simulink library "fdclib2"  (Simulink 2.09)
values from neighbouring files (symbols this model uses):
  GM1 = [cbar b    S    Ix   Iy   Iz   Jxy  Jxz  Jyz  m]    [modbuild.m]

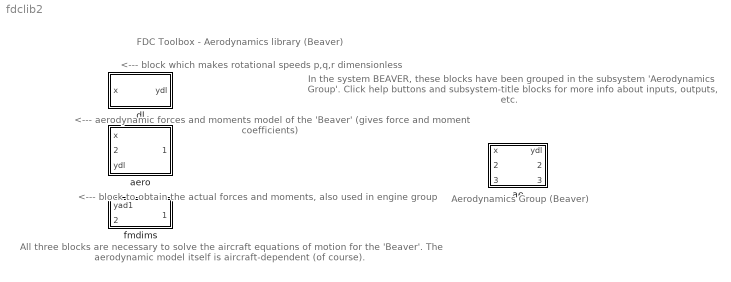
== system fdclib2 ==
  note: <--- block to obtain the actual
      | forces and moments, also used
      | in engine group
  note: <--- aerodynamic forces and moments
      | model of the 'Beaver' (gives force
      | and moment coefficients)
  note: <--- block which makes rotational
      | speeds p,q,r dimensionless
  note: All three blocks are necessary to solve the aircraft
      | equations of motion for the 'Beaver'. The aerodynamic
      | model itself is aircraft-dependent (of course).
  note: In the system BEAVER, these blocks have been
      | grouped in the subsystem 'Aerodynamics Group'.
      | Click help buttons and subsystem-title blocks
      | for more info about inputs, outputs, etc.
  note: Aerodynamics
      | Group (Beaver)
  note: FDC Toolbox - Aerodynamics library (Beaver)
  ae : Subsystem
  aero : Subsystem
      mask Type: Aeromod
      mask Description: Aerodynamic model of the DHC-2 'Beaver'.
      mask Help: eval('fdchelp aeromod')
      mask Display: disp('Aeromod\n(Beaver)')
  dl : Subsystem  mask(Dimless){cbar=GM1(1), b=GM1(2)}
      mask prompts: cbar "Mean aerodynamic chord [m]:"; b "Wing span [m]:"
      mask help: Dimensionless rotational velocities.
      mask Help: eval('fdchelp dimless')
      mask Display: disp('Dimless')
  fmdims : Subsystem  mask(FMdims){cbar=GM1(1), b=GM1(2), S=GM1(3)}
      mask prompts: cbar "Mean aerodynamic chord [m]:"; b "Wing span [m]:"; S "Wing surface [m^2]:"
      mask help:
      | Calculate forces and moments from
      | dimensionless coefficients.
      mask Help: eval('fdchelp fmdims')
      mask Display: disp('FMdims')

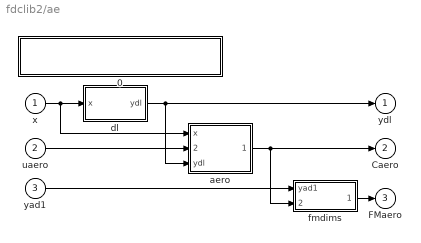
== system fdclib2/ae ==
  x : Inport  Port=1  PortWidth=-1  SampleTime=-1
  uaero : Inport  Port=2  PortWidth=-1  SampleTime=-1
  yad1 : Inport  Port=3  PortWidth=-1  SampleTime=-1
  0 : Subsystem
      settings: OpenFcn=fdchelp aerogrp
      mask Display: disp('AERODYNAMICS GROUP (level 3)\nM.O. Rauw')
  aero : Subsystem
      mask Type: Aeromod
      mask Description: Aerodynamic model of the DHC-2 'Beaver'.
      mask Help: eval('fdchelp aeromod')
      mask Display: disp('Aeromod\n(Beaver)')
  dl : Subsystem  mask(Dimless){cbar=GM1(1), b=GM1(2)}
      mask prompts: cbar "Mean aerodynamic chord [m]:"; b "Wing span [m]:"
      mask help: Dimensionless rotational velocities.
      mask Help: eval('fdchelp dimless')
      mask Display: disp('Dimless')
  fmdims : Subsystem  mask(FMdims){cbar=GM1(1), b=GM1(2), S=GM1(3)}
      mask prompts: cbar "Mean aerodynamic chord [m]:"; b "Wing span [m]:"; S "Wing surface [m^2]:"
      mask help:
      | Calculate forces and moments from
      | dimensionless coefficients.
      mask Help: eval('fdchelp fmdims')
      mask Display: disp('FMdims')
  ydl : Outport  Port=1  InitialOutput=0
  Caero : Outport  Port=2  InitialOutput=0
  FMaero : Outport  Port=3  InitialOutput=0
  wires:
  aero/1(Caero) -> Caero/1, fmdims/2(Force / moment coefficients)
  dl/1(ydl) -> ydl/1, aero/3(ydl)
  x/1 -> dl/1(x), aero/1(x)
  uaero/1 -> aero/2(uaero)
  yad1/1 -> fmdims/1(yad1)
  fmdims/1(Forces and moments) -> FMaero/1

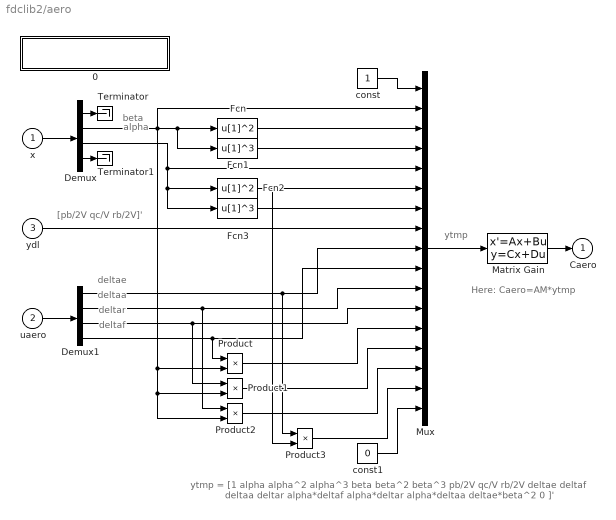
== system fdclib2/aero ==
  note: ytmp = [1  alpha  alpha^2  alpha^3  beta  beta^2  beta^3  pb/2V  qc/V  rb/2V  deltae
      | deltaf  deltaa  deltar  alpha*deltaf  alpha*deltar  alpha*deltaa  deltae*beta^2  0 ]'
  note: [pb/2V qc/V rb/2V]'
  note: beta
  note: deltae
  note: deltaa
  note: deltar
  note: deltaf
  note: alpha
  note: ytmp
  note: Here: Caero=AM*ytmp
  x : Inport  Port=1  PortWidth=-1  SampleTime=-1
  uaero : Inport  Port=2  PortWidth=-1  SampleTime=-1
  ydl : Inport  Port=3  PortWidth=-1  SampleTime=-1
  0 : Subsystem
      settings: OpenFcn=fdchelp aeromod
      mask Display: disp('AEROMOD\nM.O. Rauw, October 1997')
  Demux : Demux  Outputs=[1 1 1 9]
  Demux1 : Demux  Outputs=4
  Fcn : Fcn  Expr=u[1]^2
  Fcn1 : Fcn  Expr=u[1]^3
  Fcn2 : Fcn  Expr=u[1]^2
  Fcn3 : Fcn  Expr=u[1]^3
  Matrix Gain : StateSpace  A=A  B=B  C=C  D=D  X0=0  mask(Matrix Gain){@1=AM}
      mask prompts: @1 "Gain matrix:"
      mask help: Matrix Gain
      mask init:
      | A = []; B = []; C = []; D = @1;
      mask Help: This block implements an matrix gain.\nThe matrix dimensions must be in accordance\nwith the dimension of the inputvector.
      mask Display: disp('y = A*u')
  Mux : Mux  Inputs=[1 1 1 1 1 1 1 3 1 1 1 1 1 1 1 1 1]
  Product{,1..3} (4 alike) : Product  Inputs=2
  Terminator : Terminator
  Terminator1 : Terminator
  const : Constant  Value=1
  const1 : Constant  Value=0
  Caero : Outport  Port=1  InitialOutput=0
  wires:
  Demux/4 -> Terminator1/1
  Demux/1 -> Terminator/1
  const1/1 -> Mux/17
  const/1 -> Mux/1
  ydl/1 -> Mux/8
  Product3/1 -> Mux/16
  Product2/1 -> Mux/15
  Product1/1 -> Mux/14
  Demux1/1 -> Mux/9, Product3/1
  Fcn2/1 -> Mux/6, Product3/2
  Demux1/4 -> Mux/10, Product/1
  Demux/2 -> Mux/2, Fcn/1, Fcn1/1, Product/2, Product1/2, Product2/2
  Demux/3 -> Mux/5, Fcn2/1, Fcn3/1
  Demux1/2 -> Mux/11, Product2/1
  Demux1/3 -> Mux/12, Product1/1
  Product/1 -> Mux/13
  Fcn3/1 -> Mux/7
  uaero/1 -> Demux1/1
  Fcn1/1 -> Mux/4
  Fcn/1 -> Mux/3
  x/1 -> Demux/1
  Mux/1 -> Matrix Gain/1
  Matrix Gain/1 -> Caero/1

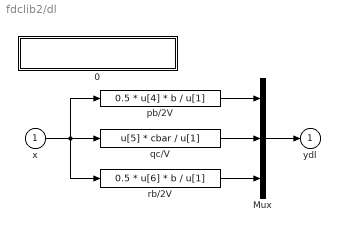
== system fdclib2/dl ==
  x : Inport  Port=1  PortWidth=-1  SampleTime=-1
  0 : Subsystem
      settings: OpenFcn=fdchelp dimless
      mask Display: disp('DIMLESS\nM.O. Rauw, October 1997')
  Mux : Mux  Inputs=3
  pb/2V : Fcn  Expr=0.5 * u[4] * b / u[1]
  qc/V : Fcn  Expr=u[5] * cbar / u[1]
  rb/2V : Fcn  Expr=0.5 * u[6] * b / u[1]
  ydl : Outport  Port=1  InitialOutput=0
  wires:
  pb/2V/1 -> Mux/1
  qc/V/1 -> Mux/2
  rb/2V/1 -> Mux/3
  Mux/1 -> ydl/1
  x/1 -> qc/V/1, rb/2V/1, pb/2V/1

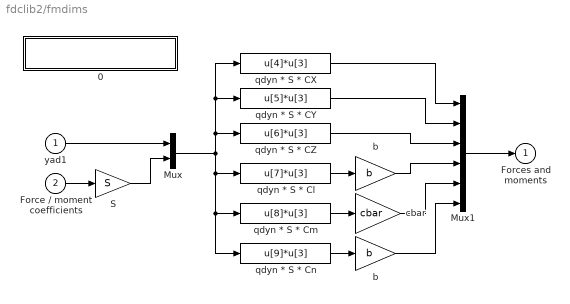
== system fdclib2/fmdims ==
  yad1 : Inport  Port=1  PortWidth=-1  SampleTime=-1
  Force / moment coefficients : Inport  Port=2  PortWidth=-1  SampleTime=-1
  0 : Subsystem
      settings: OpenFcn=fdchelp fmdims
      mask Display: disp('FMDIMS\nM.O. Rauw, October 1997')
  Mux : Mux  Inputs=[3 6]
  Mux1 : Mux  Inputs=6
  S : Gain  Gain=S
  b : Gain  Gain=b
  "b " : Gain  Gain=b
  cbar : Gain  Gain=cbar
  qdyn * S * CX : Fcn  Expr=u[4]*u[3]
  qdyn * S * CY : Fcn  Expr=u[5]*u[3]
  qdyn * S * CZ : Fcn  Expr=u[6]*u[3]
  qdyn * S * Cl : Fcn  Expr=u[7]*u[3]
  qdyn * S * Cm : Fcn  Expr=u[8]*u[3]
  qdyn * S * Cn : Fcn  Expr=u[9]*u[3]
  Forces and moments : Outport  Port=1  InitialOutput=0
  wires:
  Mux1/1 -> Forces and moments/1
  "b "/1 -> Mux1/6
  cbar/1 -> Mux1/5
  Force / moment coefficients/1 -> S/1
  Mux/1 -> qdyn * S * CZ/1, qdyn * S * CX/1, qdyn * S * CY/1, qdyn * S * Cl/1, qdyn * S * Cm/1, qdyn * S * Cn/1
  qdyn * S * Cl/1 -> b/1
  qdyn * S * Cm/1 -> cbar/1
  qdyn * S * Cn/1 -> "b "/1
  yad1/1 -> Mux/1
  qdyn * S * CX/1 -> Mux1/1
  qdyn * S * CY/1 -> Mux1/2
  S/1 -> Mux/2
  qdyn * S * CZ/1 -> Mux1/3
  b/1 -> Mux1/4

== system fdclib2/ae/0 ==

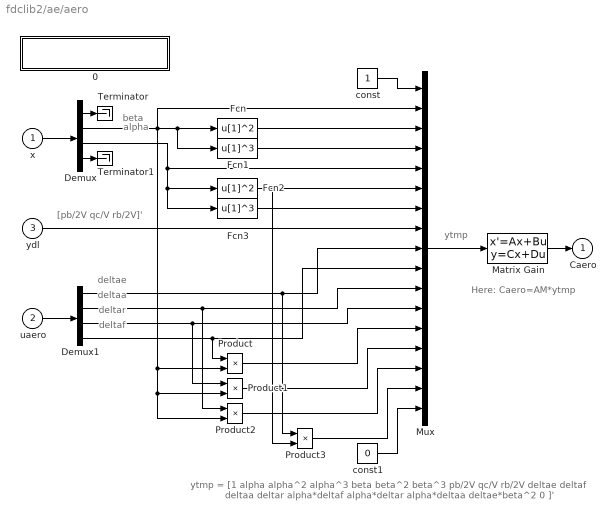
== system fdclib2/ae/aero ==
  note: ytmp = [1  alpha  alpha^2  alpha^3  beta  beta^2  beta^3  pb/2V  qc/V  rb/2V  deltae
      | deltaf  deltaa  deltar  alpha*deltaf  alpha*deltar  alpha*deltaa  deltae*beta^2  0 ]'
  note: [pb/2V qc/V rb/2V]'
  note: beta
  note: deltae
  note: deltaa
  note: deltar
  note: deltaf
  note: alpha
  note: ytmp
  note: Here: Caero=AM*ytmp
  x : Inport  Port=1  PortWidth=-1  SampleTime=-1
  uaero : Inport  Port=2  PortWidth=-1  SampleTime=-1
  ydl : Inport  Port=3  PortWidth=-1  SampleTime=-1
  0 : Subsystem
      settings: OpenFcn=fdchelp aeromod
      mask Display: disp('AEROMOD\nM.O. Rauw, October 1997')
  Demux : Demux  Outputs=[1 1 1 9]
  Demux1 : Demux  Outputs=4
  Fcn : Fcn  Expr=u[1]^2
  Fcn1 : Fcn  Expr=u[1]^3
  Fcn2 : Fcn  Expr=u[1]^2
  Fcn3 : Fcn  Expr=u[1]^3
  Matrix Gain : StateSpace  A=A  B=B  C=C  D=D  X0=0  mask(Matrix Gain){@1=AM}
      mask prompts: @1 "Gain matrix:"
      mask help: Matrix Gain
      mask init:
      | A = []; B = []; C = []; D = @1;
      mask Help: This block implements an matrix gain.\nThe matrix dimensions must be in accordance\nwith the dimension of the inputvector.
      mask Display: disp('y = A*u')
  Mux : Mux  Inputs=[1 1 1 1 1 1 1 3 1 1 1 1 1 1 1 1 1]
  Product{,1..3} (4 alike) : Product  Inputs=2
  Terminator : Terminator
  Terminator1 : Terminator
  const : Constant  Value=1
  const1 : Constant  Value=0
  Caero : Outport  Port=1  InitialOutput=0
  wires:
  Demux/4 -> Terminator1/1
  Demux/1 -> Terminator/1
  const1/1 -> Mux/17
  const/1 -> Mux/1
  ydl/1 -> Mux/8
  Product3/1 -> Mux/16
  Product2/1 -> Mux/15
  Product1/1 -> Mux/14
  Demux1/1 -> Mux/9, Product3/1
  Fcn2/1 -> Mux/6, Product3/2
  Demux1/4 -> Mux/10, Product/1
  Demux/2 -> Mux/2, Fcn/1, Fcn1/1, Product/2, Product1/2, Product2/2
  Demux/3 -> Mux/5, Fcn2/1, Fcn3/1
  Demux1/2 -> Mux/11, Product2/1
  Demux1/3 -> Mux/12, Product1/1
  Product/1 -> Mux/13
  Fcn3/1 -> Mux/7
  uaero/1 -> Demux1/1
  Fcn1/1 -> Mux/4
  Fcn/1 -> Mux/3
  x/1 -> Demux/1
  Mux/1 -> Matrix Gain/1
  Matrix Gain/1 -> Caero/1

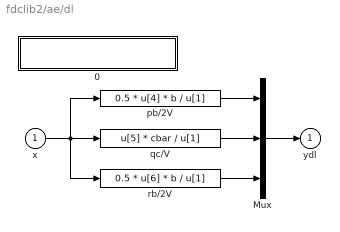
== system fdclib2/ae/dl ==
  x : Inport  Port=1  PortWidth=-1  SampleTime=-1
  0 : Subsystem
      settings: OpenFcn=fdchelp dimless
      mask Display: disp('DIMLESS\nM.O. Rauw, October 1997')
  Mux : Mux  Inputs=3
  pb/2V : Fcn  Expr=0.5 * u[4] * b / u[1]
  qc/V : Fcn  Expr=u[5] * cbar / u[1]
  rb/2V : Fcn  Expr=0.5 * u[6] * b / u[1]
  ydl : Outport  Port=1  InitialOutput=0
  wires:
  pb/2V/1 -> Mux/1
  qc/V/1 -> Mux/2
  rb/2V/1 -> Mux/3
  Mux/1 -> ydl/1
  x/1 -> qc/V/1, rb/2V/1, pb/2V/1

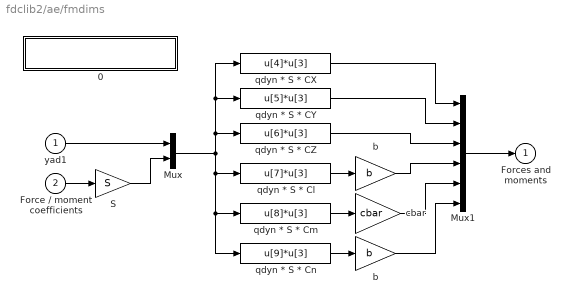
== system fdclib2/ae/fmdims ==
  yad1 : Inport  Port=1  PortWidth=-1  SampleTime=-1
  Force / moment coefficients : Inport  Port=2  PortWidth=-1  SampleTime=-1
  0 : Subsystem
      settings: OpenFcn=fdchelp fmdims
      mask Display: disp('FMDIMS\nM.O. Rauw, October 1997')
  Mux : Mux  Inputs=[3 6]
  Mux1 : Mux  Inputs=6
  S : Gain  Gain=S
  b : Gain  Gain=b
  "b " : Gain  Gain=b
  cbar : Gain  Gain=cbar
  qdyn * S * CX : Fcn  Expr=u[4]*u[3]
  qdyn * S * CY : Fcn  Expr=u[5]*u[3]
  qdyn * S * CZ : Fcn  Expr=u[6]*u[3]
  qdyn * S * Cl : Fcn  Expr=u[7]*u[3]
  qdyn * S * Cm : Fcn  Expr=u[8]*u[3]
  qdyn * S * Cn : Fcn  Expr=u[9]*u[3]
  Forces and moments : Outport  Port=1  InitialOutput=0
  wires:
  Mux1/1 -> Forces and moments/1
  "b "/1 -> Mux1/6
  cbar/1 -> Mux1/5
  Force / moment coefficients/1 -> S/1
  Mux/1 -> qdyn * S * CZ/1, qdyn * S * CX/1, qdyn * S * CY/1, qdyn * S * Cl/1, qdyn * S * Cm/1, qdyn * S * Cn/1
  qdyn * S * Cl/1 -> b/1
  qdyn * S * Cm/1 -> cbar/1
  qdyn * S * Cn/1 -> "b "/1
  yad1/1 -> Mux/1
  qdyn * S * CX/1 -> Mux1/1
  qdyn * S * CY/1 -> Mux1/2
  S/1 -> Mux/2
  qdyn * S * CZ/1 -> Mux1/3
  b/1 -> Mux1/4

== system fdclib2/aero/0 ==

== system fdclib2/dl/0 ==

== system fdclib2/fmdims/0 ==

== system fdclib2/ae/aero/0 ==

== system fdclib2/ae/dl/0 ==

== system fdclib2/ae/fmdims/0 ==
